simulink model "Expt_4_2"  (R2018a)
settings: Solver=VariableStepAuto  StartTime=0.0  StopTime=10.0  RelTol=1e-3
libraries: simulink x1
settings Model: Creator=HP  LastModifiedBy=HP

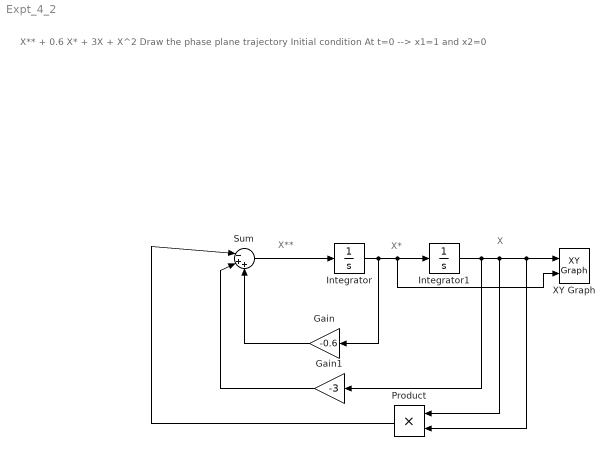
== system Expt_4_2 ==
  note: X
  note: X*
  note: X**
  note: X** + 0.6 X* + 3X + X^2
      | Draw the phase plane trajectory
      | Initial condition At t=0 --> x1=1 and x2=0
  Gain : Gain  Gain=-0.6
  Gain1 : Gain  Gain=-3
  Integrator : Integrator
  Integrator1 : Integrator  InitialCondition=1
  Product : Product
  Sum : Sum  Inputs=|-++
  XY Graph : simulink/Sinks/XY Graph  xmin=-5  xmax=5  ymin=-5  ymax=5  st=-1
  wires:
  Sum/1 -> Integrator/1
  Product/1 -> Sum/1
  Integrator1/1 -> Gain1/1, Product/1, Product/2, XY Graph/1
  Gain/1 -> Sum/3
  Gain1/1 -> Sum/2
  Integrator/1 -> Gain/1, XY Graph/2, Integrator1/1
